simulink model "Simulink_Example"  (R2025b)
settings: Solver=VariableStepAuto  StartTime=0.0  StopTime=10.0  RelTol=1e-3
settings Model: DataDictionary=Dummy_dict.sldd  Creator=georg  LastModifiedBy=georg

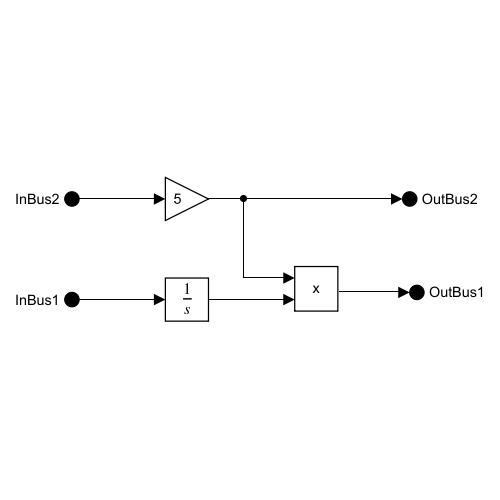
[thumbnail: Simulink's stored preview of the top-level diagram]
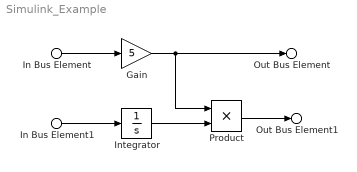
== system Simulink_Example ==
  In Bus Element : Inport  PortName=InBus2
  In Bus Element1 : Inport  Port=2  PortName=InBus1
  Gain : Gain  Gain=5
  Integrator : Integrator
  Product : Product
  Out Bus Element : Outport  PortName=OutBus2
  Out Bus Element1 : Outport  Port=2  PortName=OutBus1
  wires:
  In Bus Element/1 -> Gain/1
  Gain/1 -> Product/1, Out Bus Element/1
  In Bus Element1/1 -> Integrator/1
  Integrator/1 -> Product/2
  Product/1 -> Out Bus Element1/1
